simulink model "rfsignalgenerator"  (R2020a)
settings: Solver=VariableStepAuto  StartTime=0.0  StopTime=inf  RelTol=1e-3
InitFcn:
  | run ./scripts/rfgen.m
undefined symbols (not defined in the file): fs
libraries: dspswit3 x2, lib_rfsignalgenerator x1
settings Model: Creator=lewisdav  LastModifiedBy=LDM
settings SFSimCC: CustomCodeUndefinedFunction=UseInterfaceOnly

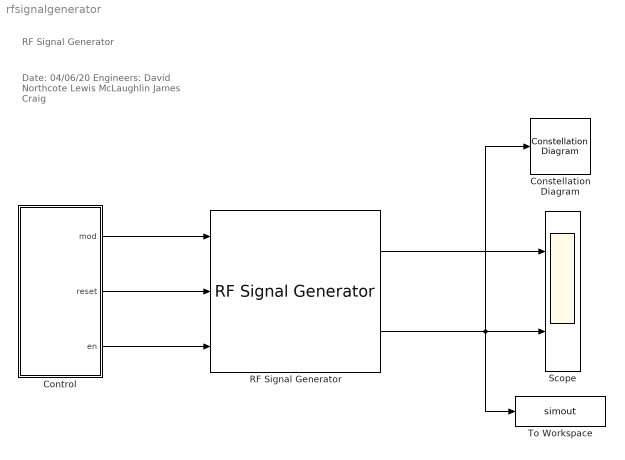
== system rfsignalgenerator ==
  note: RF Signal Generator
  note: Date: 04/06/20
      | Engineers: David Northcote
      | Lewis McLaughlin
      | James Craig
  Constellation Diagram : ConstellationDiagram
  Control : Subsystem  mask{mod_mask=1024QAM, en=on}
      mask prompts: mod_mask "Modulation"; en "Enable"
      mask init:
      | % RF Signal Generator
      | if strcmpi(get_param(gcb, 'mod_mask'), 'BPSK')
      |     mod = 0;
      | elseif strcmpi(get_param(gcb, 'mod_mask'), 'QPSK')
      |     mod = 1;
      | elseif strcmpi(get_param(gcb, 'mod_mask'), '8PSK')
      |     mod = 2;
      | elseif strcmpi(get_param(gcb, 'mod_mask'), '16QAM')
      |     mod = 3;
      | elseif strcmpi(get_param(gcb, 'mod_mask'), '32QAM')
      |     mod = 4;
      | elseif strcmpi(get_param(gcb, 'mod_mask'), '64QAM')
      |     mod = 5;
      | elseif strcmpi(get_param(gcb, 'mod_mask'), '128QAM')
      |     mod = 6;
      | elseif strcmpi(get_param(gcb, 'mod_mask'), '256QAM')
      |     mod = 7;
      | elseif strcmpi(get_param(gcb, 'mod_mask'), '512QAM')
      |     mod = 8;
      | elseif strcmpi(get_param(gcb, 'mod_mask'), '1024QAM')
      |     mod = 9;
      | end
      mask TypeOptions mod_mask: BPSK | QPSK | 8PSK | 16QAM | 32QAM | 64QAM | 128QAM | 256QAM | 512QAM | 1024QAM
      mask DialogControl DescGroupVar Prompt: RF Signal Generator
      mask DialogControl DescTextVar Prompt: Exposes parameters the user can control from Jupyter when running on the target.
      mask DialogControl Container3 Prompt: Control
      mask DialogControl reset Prompt: Reset
      mask DialogControl reset Callback:
      | x = get_param(sprintf('%s/trans_reset', gcb), 'value');
      | 
      | if x == '1'
      |     set_param(sprintf('%s/trans_reset', gcb), 'value', '0')
      | else
      |     set_param(sprintf('%s/trans_reset', gcb), 'value', '1')
      | end
  RF Signal Generator : lib_rfsignalgenerator/RF Signal Generator  SystemSampleTime=-1  Latency=0  AutoFrameSizeCalculation=off
  Scope : Scope  NumInputPorts=2
  To Workspace : ToWorkspace  VariableName=simout  SampleTime=-1
      settings: MaxDataPoints=8192  Save2DSignal=2-D array (concatenate along first dimension)
  wires:
  Control/2(reset) -> RF Signal Generator/2
  Control/1(mod) -> RF Signal Generator/1
  Control/3(en) -> RF Signal Generator/3
  RF Signal Generator/2 -> Scope/2, To Workspace/1, Constellation Diagram/1
  RF Signal Generator/1 -> Scope/1

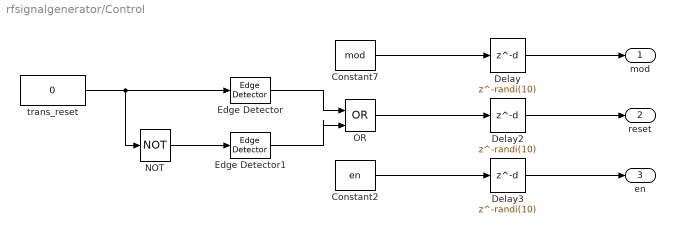
== system rfsignalgenerator/Control ==
  Constant2 : Constant  Value=en  OutDataTypeStr=boolean  SampleTime=1/fs
  Constant7 : Constant  Value=mod  VectorParams1D=off  OutDataTypeStr=uint32  SampleTime=1/fs
  Delay : Delay  DelayLength=randi(10)
  Delay2 : Delay  DelayLength=randi(10)
  Delay3 : Delay  DelayLength=randi(10)
  Edge Detector : dspswit3/Edge Detector  InputProcessing=Columns as channels (frame based)
      settings: SourceProductBaseCode=DS
  Edge Detector1 : dspswit3/Edge Detector  InputProcessing=Columns as channels (frame based)
      settings: SourceProductBaseCode=DS
  NOT : Logic  Operator=NOT  IconShape=distinctive  AllPortsSameDT=off  OutDataTypeStr=boolean
  OR : Logic  Operator=OR  IconShape=distinctive  AllPortsSameDT=off  OutDataTypeStr=boolean
  trans_reset : Constant  Value=0  OutDataTypeStr=boolean  SampleTime=1/fs
  mod : Outport  VectorParamsAs1DForOutWhenUnconnected=off
  reset : Outport  Port=2  VectorParamsAs1DForOutWhenUnconnected=off
  en : Outport  Port=3  VectorParamsAs1DForOutWhenUnconnected=off
  wires:
  trans_reset/1 -> NOT/1, Edge Detector/1
  NOT/1 -> Edge Detector1/1
  Edge Detector/1 -> OR/1
  Edge Detector1/1 -> OR/2
  Delay3/1 -> en/1
  Delay2/1 -> reset/1
  OR/1 -> Delay2/1
  Delay/1 -> mod/1
  Constant7/1 -> Delay/1
  Constant2/1 -> Delay3/1
